simulink model "PID"  (R2024b)
settings: Solver=VariableStepAuto  StartTime=0.0  StopTime=t_sim  RelTol=1e-3
values from neighbouring files (symbols this model uses):
  Ax = [0 1; 0 0]    [Main_PID.m]
  Ay = [0 1; 0 0]    [Main_PID.m]
  b = 0.0245    [Main_PID.m]
  Bx = [0 Cx]'    [Main_PID.m]
  By = [0 Cy]'    [Main_PID.m]
  CCx = [1 0]    [Main_PID.m]
  CCy = [1 0]    [Main_PID.m]
  Cx = m*g*b/(m+J/r^2)/lx    (= 0.943269230769)    [Main_PID.m]
  Cy = m*g*b/(m+J/r^2)/ly    (= 1.1445)    [Main_PID.m]
  data_sys = [m r g J b lx ly]    [Main_PID.m]
  Dx = 0    [Main_PID.m]
  Dy = 0    [Main_PID.m]
  Kb_x = 0    [Main_PID.m]
  Kb_y = 0    [Main_PID.m]
  Kd_x = 3    [Main_PID.m]
  Kd_y = Kd_x/1.2    (= 2.5)    [Main_PID.m]
  Ki_x = 5    [Main_PID.m]
  Ki_y = Ki_x/1.2    (= 4.16666666667)    [Main_PID.m]
  Kp_x = 5    [Main_PID.m]
  Kp_y = Kp_x/1.2    (= 4.16666666667)    [Main_PID.m]
  lx = 0.182    [Main_PID.m]
  ly = 0.150    (= 0.15)    [Main_PID.m]
  N_x = 15    [Main_PID.m]
  N_y = 15    [Main_PID.m]
  ux_lim = 45    [Main_PID.m]
  uy_lim = 45    [Main_PID.m]
  x_ref = 0.05    [Main_PID.m]
  y_ref = 0.05    [Main_PID.m]
  zx0 = [x0 xp0]'    [Main_PID.m]
  zy0 = [y0 yp0]'    [Main_PID.m]
libraries: slpidlib x4
settings Model: Creator=nicvi  LastModifiedBy=nicvi

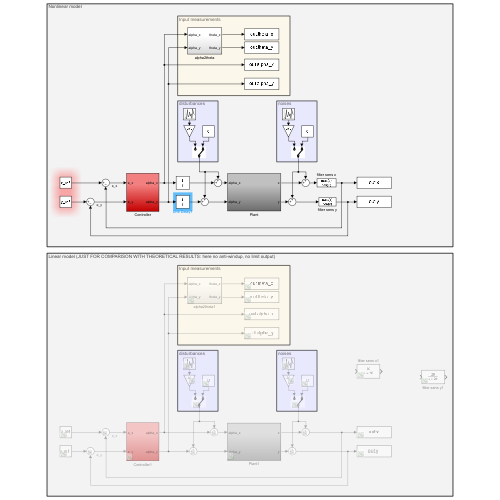
[thumbnail: Simulink's stored preview of the top-level diagram]
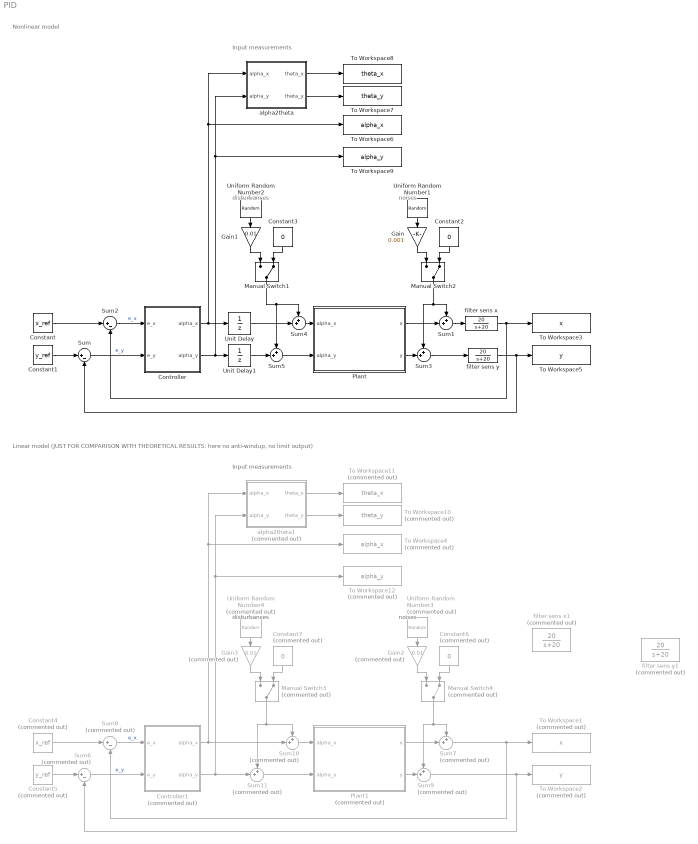
== system PID ==
  note: Nonlinear model
  note: noises
  note: Input measurements
  note: disturbances
  note: Linear model (JUST FOR COMPARISON WITH THEORETICAL RESULTS: here no anti-windup, no limit output)
  note: noises
  note: disturbances
  note: Input measurements
  Constant : Constant  Value=x_ref  SampleTime=-1
  Constant1 : Constant  Value=y_ref  SampleTime=-1
  Constant2 : Constant  Value=0
  Constant3 : Constant  Value=0
  Constant4 : Constant  Commented=on  Value=x_ref  SampleTime=-1
  Constant5 : Constant  Commented=on  Value=y_ref  SampleTime=-1
  Constant6 : Constant  Commented=on  Value=0
  Constant7 : Constant  Commented=on  Value=0
  Controller : Subsystem
  Controller1 : Subsystem  Commented=on
  Gain : Gain  Gain=0.001
  Gain1 : Gain  Gain=0.01
  Gain2 : Gain  Commented=on  Gain=0.01
  Gain3 : Gain  Commented=on  Gain=0.01
  Manual Switch1 : ManualSwitch  CurrentSetting=0
  Manual Switch2 : ManualSwitch  CurrentSetting=0
  Manual Switch3 : ManualSwitch  Commented=on  CurrentSetting=0
  Manual Switch4 : ManualSwitch  Commented=on  CurrentSetting=0
  Plant : Subsystem
  Plant1 : Subsystem  Commented=on
  Sum : Sum  Inputs=|+-
  Sum{1,3..5} (4 alike) : Sum  Inputs=++|
  Sum{7,9..11} (4 alike) : Sum  Commented=on  Inputs=++|
  Sum2 : Sum  Inputs=|+-
  Sum6 : Sum  Commented=on  Inputs=|+-
  Sum8 : Sum  Commented=on  Inputs=|+-
  To Workspace1 : ToWorkspace  Commented=on  VariableName=x  SampleTime=-1
      settings: Save2DSignal=2-D array (concatenate along first dimension)
  To Workspace10 : ToWorkspace  Commented=on  VariableName=theta_y  SampleTime=-1
      settings: Save2DSignal=2-D array (concatenate along first dimension)
  To Workspace11 : ToWorkspace  Commented=on  VariableName=theta_x  SampleTime=-1
      settings: Save2DSignal=2-D array (concatenate along first dimension)
  To Workspace12 : ToWorkspace  Commented=on  VariableName=alpha_y  SampleTime=-1
      settings: Save2DSignal=2-D array (concatenate along first dimension)
  To Workspace2 : ToWorkspace  Commented=on  VariableName=y  SampleTime=-1
      settings: Save2DSignal=2-D array (concatenate along first dimension)
  To Workspace3 : ToWorkspace  VariableName=x  SampleTime=-1
      settings: Save2DSignal=2-D array (concatenate along first dimension)
  To Workspace4 : ToWorkspace  Commented=on  VariableName=alpha_x  SampleTime=-1
      settings: Save2DSignal=2-D array (concatenate along first dimension)
  To Workspace5 : ToWorkspace  VariableName=y  SampleTime=-1
      settings: Save2DSignal=2-D array (concatenate along first dimension)
  To Workspace6 : ToWorkspace  VariableName=alpha_x  SampleTime=-1
      settings: Save2DSignal=2-D array (concatenate along first dimension)
  To Workspace7 : ToWorkspace  VariableName=theta_y  SampleTime=-1
      settings: Save2DSignal=2-D array (concatenate along first dimension)
  To Workspace8 : ToWorkspace  VariableName=theta_x  SampleTime=-1
      settings: Save2DSignal=2-D array (concatenate along first dimension)
  To Workspace9 : ToWorkspace  VariableName=alpha_y  SampleTime=-1
      settings: Save2DSignal=2-D array (concatenate along first dimension)
  Uniform Random Number1 : UniformRandomNumber  SampleTime=0.1
  Uniform Random Number2 : UniformRandomNumber  Minimum=5  Maximum=7  SampleTime=0.01
  Uniform Random Number3 : UniformRandomNumber  Commented=on  SampleTime=0.01
  Uniform Random Number4 : UniformRandomNumber  Commented=on  SampleTime=0.01
  Unit Delay : UnitDelay  SampleTime=0.08  HasFrameUpgradeWarning=on
  Unit Delay1 : UnitDelay  SampleTime=0.08  HasFrameUpgradeWarning=on
  alpha2theta : Subsystem
  alpha2theta1 : Subsystem  Commented=on
  filter sens x : TransferFcn  Numerator=[20]  Denominator=[1 20]
  filter sens x1 : TransferFcn  Commented=on  Numerator=[20]  Denominator=[1 20]
  filter sens y : TransferFcn  Numerator=[20]  Denominator=[1 20]
  filter sens y1 : TransferFcn  Commented=on  Numerator=[20]  Denominator=[1 20]
  wires:
  Constant/1 -> Sum2/1
  Constant1/1 -> Sum/1
  Sum2/1 -> Controller/1(e_x)  "e_x"
  Sum/1 -> Controller/2(e_y)  "e_y"
  Controller/1(alpha_x) -> Unit Delay/1, To Workspace6/1, alpha2theta/1(alpha_x)
  Controller/2(alpha_y) -> To Workspace9/1, alpha2theta/2(alpha_y), Unit Delay1/1
  alpha2theta/1(theta_x) -> To Workspace8/1
  alpha2theta/2(theta_y) -> To Workspace7/1
  Plant/2(y) -> Sum3/2
  Plant/1(x) -> Sum1/2
  Constant2/1 -> Manual Switch2/2
  Uniform Random Number1/1 -> Gain/1
  Gain/1 -> Manual Switch2/1
  Manual Switch2/1 -> Sum1/1, Sum3/1
  Manual Switch1/1 -> Sum5/1, Sum4/1
  Constant3/1 -> Manual Switch1/2
  Gain1/1 -> Manual Switch1/1
  Uniform Random Number2/1 -> Gain1/1
  Sum4/1 -> Plant/1(alpha_x)
  Sum5/1 -> Plant/2(alpha_y)
  Uniform Random Number3/1 -> Gain2/1
  Sum10/1 -> Plant1/1(alpha_x)
  Manual Switch3/1 -> Sum11/1, Sum10/1
  alpha2theta1/1(theta_x) -> To Workspace11/1
  Sum8/1 -> Controller1/1(e_x)  "e_x"
  Constant5/1 -> Sum6/1
  Controller1/2(alpha_y) -> Sum11/2, To Workspace12/1, alpha2theta1/2(alpha_y)
  Sum11/1 -> Plant1/2(alpha_y)
  Controller1/1(alpha_x) -> Sum10/2, To Workspace4/1, alpha2theta1/1(alpha_x)
  Constant4/1 -> Sum8/1
  Sum6/1 -> Controller1/2(e_y)  "e_y"
  Constant7/1 -> Manual Switch3/2
  Manual Switch4/1 -> Sum7/1, Sum9/1
  alpha2theta1/2(theta_y) -> To Workspace10/1
  Plant1/2(y) -> Sum9/2
  Sum9/1 -> To Workspace2/1, Sum6/2
  Gain2/1 -> Manual Switch4/1
  Gain3/1 -> Manual Switch3/1
  Uniform Random Number4/1 -> Gain3/1
  Constant6/1 -> Manual Switch4/2
  Sum7/1 -> To Workspace1/1, Sum8/2
  Plant1/1(x) -> Sum7/2
  Sum1/1 -> filter sens x/1
  Sum3/1 -> filter sens y/1
  filter sens x/1 -> To Workspace3/1, Sum2/2
  filter sens y/1 -> To Workspace5/1, Sum/2
  Unit Delay/1 -> Sum4/2
  Unit Delay1/1 -> Sum5/2

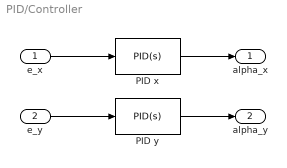
== system PID/Controller ==
  e_x : Inport
  e_y : Inport  Port=2
  PID x : slpidlib/PID Controller  Controller=PID  Form=Parallel  TimeDomain=Continuous-time  UseExternalTs=off  SampleTime=-1  IntegratorMethod=Forward Euler  FilterMethod=Forward Euler  ControllerParametersSource=internal  P=Kp_x  I=Ki_x  UseKiTs=off  D=Kd_x  UseExternalDerivativeSource=off  N=N_x  UseFilter=on  TunerSelectOption=Transfer Function Based (PID Tuner App)  InitialConditionSource=internal  InitialConditionForIntegrator=0  InitialConditionForFilter=0  DifferentiatorICPrevScaledInput=0  ExternalReset=none  TrackingMode=off  Kt=1  LimitOutput=on  SatLimitsSource=internal  UpperSaturationLimit=deg2rad(ux_lim)  LowerSaturationLimit=deg2rad(-ux_lim)  LinearizeAsGain=on  AntiWindupMode=back-calculation  Kb=Kb_x  LimitIntegrator=off  UpperIntegratorSaturationLimit=inf  LowerIntegratorSaturationLimit=-inf  POutMin=[]  POutMax=[]  IOutMin=[]  IOutMax=[]  DOutMin=[]  DOutMax=[]  NOutMin=[]  NOutMax=[]  SumOutMin=[]  SumOutMax=[]  SaturationOutMin=[]  SaturationOutMax=[]  PParamMin=[]  PParamMax=[]  IParamMin=[]  IParamMax=[]  DParamMin=[]  DParamMax=[]  NParamMin=[]  NParamMax=[]  KbParamMin=[]  KbParamMax=[]  KtParamMin=[]  KtParamMax=[]  KbOutMin=[]  KbOutMax=[]  KtOutMin=[]  KtOutMax=[]  IntegratorOutMin=[]  IntegratorOutMax=[]  FilterOutMin=[]  FilterOutMax=[]  SumI1OutMin=[]  SumI1OutMax=[]  SumI2OutMin=[]  SumI2OutMax=[]  SumI3OutMin=[]  SumI3OutMax=[]  SumI4OutMin=[]  SumI4OutMax=[]  SumDOutMin=[]  SumDOutMax=[]  DifferentiatorOutMin=[]  DifferentiatorOutMax=[]  FilterDiffOutCoefMin=[]  FilterDiffOutCoefMax=[]  ReciprocalOutMin=[]  ReciprocalOutMax=[]  SumDenOutMin=[]  SumDenOutMax=[]  SumNumOutMin=[]  SumNumOutMax=[]  DivideOutMin=[]  DivideOutMax=[]  UdiffTsProdOutMin=[]  UdiffTsProdOutMax=[]  NTsProdOutMin=[]  NTsProdOutMax=[]  UintegralTsProdOutMin=[]  UintegralTsProdOutMax=[]  UngainTsProdOutMin=[]  UngainTsProdOutMax=[]  ClampingZeroOutDataTypeStr=Inherit: Inherit via back propagation  ClampingZeroOutMin=[]  ClampingZeroOutMax=[]  FilterDenConstantOutDataTypeStr=Inherit: Inherit via back propagation  FilterDenConstantOutMin=[]  FilterDenConstantOutMax=[]  PCopyOutDataTypeStr=Inherit: Inherit via back propagation  PCopyOutMin=[]  PCopyOutMax=[]  NCopyOutDataTypeStr=Inherit: Inherit via back propagation  NCopyOutMin=[]  NCopyOutMax=[]  IntegratorContinuousStateAttributes=''  IntegratorStateMustResolveToSignalObject=off  IntegratorRTWStateStorageClass=Auto  FilterContinuousStateAttributes=''  FilterStateMustResolveToSignalObject=off  FilterRTWStateStorageClass=Auto  ParallelPVariant=InternalParameters  IdealPVariant=Disabled  IVariant=InternalParameters  DVariant=InternalParameters  IntegratorVariant=Continuous  SatVariant=Enabled  AWVariant=BackCalculation  PCopyVariant=Disabled  TRVariant=Disabled  FdbkBlocksVariant=Forward  IdealPFdbkVariant=Disabled  SatFdbkVariant=Disabled  DerivativeFilterVariant=ContFilter  NVariant=InternalParameters  NCopyVariant=Disabled  FilterICVariant=InternalICsFilter  IntegratorICVariant=InternalICs  ExternalResetVariant=Disabled  TRSumVariant=Passthrough  SumFdbkVariant=Disabled  SumVariant=Sum_PID  TsampFilterVariant=InternalTs  TsampNgainVariant=Passthrough  TsampIntegralVariant=Disabled_SignalSpec  ExternalSaturationOutDataTypeStr=Inherit: Same as second input  DerivativeSourceVariant=ErrorSignal  PreIntVariant=InternalPreInt
  PID y : slpidlib/PID Controller  Controller=PID  Form=Parallel  TimeDomain=Continuous-time  UseExternalTs=off  SampleTime=-1  IntegratorMethod=Forward Euler  FilterMethod=Forward Euler  ControllerParametersSource=internal  P=Kp_y  I=Ki_y  UseKiTs=off  D=Kd_y  UseExternalDerivativeSource=off  N=N_y  UseFilter=on  TunerSelectOption=Transfer Function Based (PID Tuner App)  InitialConditionSource=internal  InitialConditionForIntegrator=0  InitialConditionForFilter=0  DifferentiatorICPrevScaledInput=0  ExternalReset=none  TrackingMode=off  Kt=1  LimitOutput=on  SatLimitsSource=internal  UpperSaturationLimit=deg2rad(uy_lim)  LowerSaturationLimit=deg2rad(-uy_lim)  LinearizeAsGain=on  AntiWindupMode=back-calculation  Kb=Kb_y  LimitIntegrator=off  UpperIntegratorSaturationLimit=inf  LowerIntegratorSaturationLimit=-inf  POutMin=[]  POutMax=[]  IOutMin=[]  IOutMax=[]  DOutMin=[]  DOutMax=[]  NOutMin=[]  NOutMax=[]  SumOutMin=[]  SumOutMax=[]  SaturationOutMin=[]  SaturationOutMax=[]  PParamMin=[]  PParamMax=[]  IParamMin=[]  IParamMax=[]  DParamMin=[]  DParamMax=[]  NParamMin=[]  NParamMax=[]  KbParamMin=[]  KbParamMax=[]  KtParamMin=[]  KtParamMax=[]  KbOutMin=[]  KbOutMax=[]  KtOutMin=[]  KtOutMax=[]  IntegratorOutMin=[]  IntegratorOutMax=[]  FilterOutMin=[]  FilterOutMax=[]  SumI1OutMin=[]  SumI1OutMax=[]  SumI2OutMin=[]  SumI2OutMax=[]  SumI3OutMin=[]  SumI3OutMax=[]  SumI4OutMin=[]  SumI4OutMax=[]  SumDOutMin=[]  SumDOutMax=[]  DifferentiatorOutMin=[]  DifferentiatorOutMax=[]  FilterDiffOutCoefMin=[]  FilterDiffOutCoefMax=[]  ReciprocalOutMin=[]  ReciprocalOutMax=[]  SumDenOutMin=[]  SumDenOutMax=[]  SumNumOutMin=[]  SumNumOutMax=[]  DivideOutMin=[]  DivideOutMax=[]  UdiffTsProdOutMin=[]  UdiffTsProdOutMax=[]  NTsProdOutMin=[]  NTsProdOutMax=[]  UintegralTsProdOutMin=[]  UintegralTsProdOutMax=[]  UngainTsProdOutMin=[]  UngainTsProdOutMax=[]  ClampingZeroOutDataTypeStr=Inherit: Inherit via back propagation  ClampingZeroOutMin=[]  ClampingZeroOutMax=[]  FilterDenConstantOutDataTypeStr=Inherit: Inherit via back propagation  FilterDenConstantOutMin=[]  FilterDenConstantOutMax=[]  PCopyOutDataTypeStr=Inherit: Inherit via back propagation  PCopyOutMin=[]  PCopyOutMax=[]  NCopyOutDataTypeStr=Inherit: Inherit via back propagation  NCopyOutMin=[]  NCopyOutMax=[]  IntegratorContinuousStateAttributes=''  IntegratorStateMustResolveToSignalObject=off  IntegratorRTWStateStorageClass=Auto  FilterContinuousStateAttributes=''  FilterStateMustResolveToSignalObject=off  FilterRTWStateStorageClass=Auto  ParallelPVariant=InternalParameters  IdealPVariant=Disabled  IVariant=InternalParameters  DVariant=InternalParameters  IntegratorVariant=Continuous  SatVariant=Enabled  AWVariant=BackCalculation  PCopyVariant=Disabled  TRVariant=Disabled  FdbkBlocksVariant=Forward  IdealPFdbkVariant=Disabled  SatFdbkVariant=Disabled  DerivativeFilterVariant=ContFilter  NVariant=InternalParameters  NCopyVariant=Disabled  FilterICVariant=InternalICsFilter  IntegratorICVariant=InternalICs  ExternalResetVariant=Disabled  TRSumVariant=Passthrough  SumFdbkVariant=Disabled  SumVariant=Sum_PID  TsampFilterVariant=InternalTs  TsampNgainVariant=Passthrough  TsampIntegralVariant=Disabled_SignalSpec  ExternalSaturationOutDataTypeStr=Inherit: Same as second input  DerivativeSourceVariant=ErrorSignal  PreIntVariant=InternalPreInt
  alpha_x : Outport
  alpha_y : Outport  Port=2
  wires:
  PID y/1 -> alpha_y/1
  e_y/1 -> PID y/1
  e_x/1 -> PID x/1
  PID x/1 -> alpha_x/1

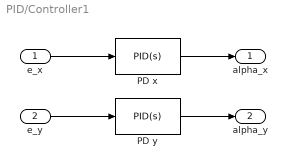
== system PID/Controller1 ==
  e_x : Inport
  e_y : Inport  Port=2
  PD x : slpidlib/PID Controller  Controller=PID  Form=Parallel  TimeDomain=Continuous-time  UseExternalTs=off  SampleTime=-1  IntegratorMethod=Forward Euler  FilterMethod=Forward Euler  ControllerParametersSource=internal  P=Kp_x  I=Ki_x  UseKiTs=off  D=Kd_x  UseExternalDerivativeSource=off  N=N_x  UseFilter=on  TunerSelectOption=Transfer Function Based (PID Tuner App)  InitialConditionSource=internal  InitialConditionForIntegrator=0  InitialConditionForFilter=0  DifferentiatorICPrevScaledInput=0  ExternalReset=none  TrackingMode=off  Kt=1  LimitOutput=on  SatLimitsSource=internal  UpperSaturationLimit=deg2rad(ux_lim)  LowerSaturationLimit=deg2rad(-ux_lim)  LinearizeAsGain=on  AntiWindupMode=back-calculation  Kb=Kb_x  LimitIntegrator=off  UpperIntegratorSaturationLimit=inf  LowerIntegratorSaturationLimit=-inf  POutMin=[]  POutMax=[]  IOutMin=[]  IOutMax=[]  DOutMin=[]  DOutMax=[]  NOutMin=[]  NOutMax=[]  SumOutMin=[]  SumOutMax=[]  SaturationOutMin=[]  SaturationOutMax=[]  PParamMin=[]  PParamMax=[]  IParamMin=[]  IParamMax=[]  DParamMin=[]  DParamMax=[]  NParamMin=[]  NParamMax=[]  KbParamMin=[]  KbParamMax=[]  KtParamMin=[]  KtParamMax=[]  KbOutMin=[]  KbOutMax=[]  KtOutMin=[]  KtOutMax=[]  IntegratorOutMin=[]  IntegratorOutMax=[]  FilterOutMin=[]  FilterOutMax=[]  SumI1OutMin=[]  SumI1OutMax=[]  SumI2OutMin=[]  SumI2OutMax=[]  SumI3OutMin=[]  SumI3OutMax=[]  SumI4OutMin=[]  SumI4OutMax=[]  SumDOutMin=[]  SumDOutMax=[]  DifferentiatorOutMin=[]  DifferentiatorOutMax=[]  FilterDiffOutCoefMin=[]  FilterDiffOutCoefMax=[]  ReciprocalOutMin=[]  ReciprocalOutMax=[]  SumDenOutMin=[]  SumDenOutMax=[]  SumNumOutMin=[]  SumNumOutMax=[]  DivideOutMin=[]  DivideOutMax=[]  UdiffTsProdOutMin=[]  UdiffTsProdOutMax=[]  NTsProdOutMin=[]  NTsProdOutMax=[]  UintegralTsProdOutMin=[]  UintegralTsProdOutMax=[]  UngainTsProdOutMin=[]  UngainTsProdOutMax=[]  ClampingZeroOutDataTypeStr=Inherit: Inherit via back propagation  ClampingZeroOutMin=[]  ClampingZeroOutMax=[]  FilterDenConstantOutDataTypeStr=Inherit: Inherit via back propagation  FilterDenConstantOutMin=[]  FilterDenConstantOutMax=[]  PCopyOutDataTypeStr=Inherit: Inherit via back propagation  PCopyOutMin=[]  PCopyOutMax=[]  NCopyOutDataTypeStr=Inherit: Inherit via back propagation  NCopyOutMin=[]  NCopyOutMax=[]  IntegratorContinuousStateAttributes=''  IntegratorStateMustResolveToSignalObject=off  IntegratorRTWStateStorageClass=Auto  FilterContinuousStateAttributes=''  FilterStateMustResolveToSignalObject=off  FilterRTWStateStorageClass=Auto  ParallelPVariant=InternalParameters  IdealPVariant=Disabled  IVariant=InternalParameters  DVariant=InternalParameters  IntegratorVariant=Continuous  SatVariant=Enabled  AWVariant=BackCalculation  PCopyVariant=Disabled  TRVariant=Disabled  FdbkBlocksVariant=Forward  IdealPFdbkVariant=Disabled  SatFdbkVariant=Disabled  DerivativeFilterVariant=ContFilter  NVariant=InternalParameters  NCopyVariant=Disabled  FilterICVariant=InternalICsFilter  IntegratorICVariant=InternalICs  ExternalResetVariant=Disabled  TRSumVariant=Passthrough  SumFdbkVariant=Disabled  SumVariant=Sum_PID  TsampFilterVariant=InternalTs  TsampNgainVariant=Passthrough  TsampIntegralVariant=Disabled_SignalSpec  ExternalSaturationOutDataTypeStr=Inherit: Same as second input  DerivativeSourceVariant=ErrorSignal  PreIntVariant=InternalPreInt
  PD y : slpidlib/PID Controller  Controller=PID  Form=Parallel  TimeDomain=Continuous-time  UseExternalTs=off  SampleTime=-1  IntegratorMethod=Forward Euler  FilterMethod=Forward Euler  ControllerParametersSource=internal  P=Kp_y  I=Ki_y  UseKiTs=off  D=Kd_y  UseExternalDerivativeSource=off  N=N_y  UseFilter=on  TunerSelectOption=Transfer Function Based (PID Tuner App)  InitialConditionSource=internal  InitialConditionForIntegrator=0  InitialConditionForFilter=0  DifferentiatorICPrevScaledInput=0  ExternalReset=none  TrackingMode=off  Kt=1  LimitOutput=on  SatLimitsSource=internal  UpperSaturationLimit=deg2rad(uy_lim)  LowerSaturationLimit=deg2rad(-uy_lim)  LinearizeAsGain=on  AntiWindupMode=back-calculation  Kb=Kb_y  LimitIntegrator=off  UpperIntegratorSaturationLimit=inf  LowerIntegratorSaturationLimit=-inf  POutMin=[]  POutMax=[]  IOutMin=[]  IOutMax=[]  DOutMin=[]  DOutMax=[]  NOutMin=[]  NOutMax=[]  SumOutMin=[]  SumOutMax=[]  SaturationOutMin=[]  SaturationOutMax=[]  PParamMin=[]  PParamMax=[]  IParamMin=[]  IParamMax=[]  DParamMin=[]  DParamMax=[]  NParamMin=[]  NParamMax=[]  KbParamMin=[]  KbParamMax=[]  KtParamMin=[]  KtParamMax=[]  KbOutMin=[]  KbOutMax=[]  KtOutMin=[]  KtOutMax=[]  IntegratorOutMin=[]  IntegratorOutMax=[]  FilterOutMin=[]  FilterOutMax=[]  SumI1OutMin=[]  SumI1OutMax=[]  SumI2OutMin=[]  SumI2OutMax=[]  SumI3OutMin=[]  SumI3OutMax=[]  SumI4OutMin=[]  SumI4OutMax=[]  SumDOutMin=[]  SumDOutMax=[]  DifferentiatorOutMin=[]  DifferentiatorOutMax=[]  FilterDiffOutCoefMin=[]  FilterDiffOutCoefMax=[]  ReciprocalOutMin=[]  ReciprocalOutMax=[]  SumDenOutMin=[]  SumDenOutMax=[]  SumNumOutMin=[]  SumNumOutMax=[]  DivideOutMin=[]  DivideOutMax=[]  UdiffTsProdOutMin=[]  UdiffTsProdOutMax=[]  NTsProdOutMin=[]  NTsProdOutMax=[]  UintegralTsProdOutMin=[]  UintegralTsProdOutMax=[]  UngainTsProdOutMin=[]  UngainTsProdOutMax=[]  ClampingZeroOutDataTypeStr=Inherit: Inherit via back propagation  ClampingZeroOutMin=[]  ClampingZeroOutMax=[]  FilterDenConstantOutDataTypeStr=Inherit: Inherit via back propagation  FilterDenConstantOutMin=[]  FilterDenConstantOutMax=[]  PCopyOutDataTypeStr=Inherit: Inherit via back propagation  PCopyOutMin=[]  PCopyOutMax=[]  NCopyOutDataTypeStr=Inherit: Inherit via back propagation  NCopyOutMin=[]  NCopyOutMax=[]  IntegratorContinuousStateAttributes=''  IntegratorStateMustResolveToSignalObject=off  IntegratorRTWStateStorageClass=Auto  FilterContinuousStateAttributes=''  FilterStateMustResolveToSignalObject=off  FilterRTWStateStorageClass=Auto  ParallelPVariant=InternalParameters  IdealPVariant=Disabled  IVariant=InternalParameters  DVariant=InternalParameters  IntegratorVariant=Continuous  SatVariant=Enabled  AWVariant=BackCalculation  PCopyVariant=Disabled  TRVariant=Disabled  FdbkBlocksVariant=Forward  IdealPFdbkVariant=Disabled  SatFdbkVariant=Disabled  DerivativeFilterVariant=ContFilter  NVariant=InternalParameters  NCopyVariant=Disabled  FilterICVariant=InternalICsFilter  IntegratorICVariant=InternalICs  ExternalResetVariant=Disabled  TRSumVariant=Passthrough  SumFdbkVariant=Disabled  SumVariant=Sum_PID  TsampFilterVariant=InternalTs  TsampNgainVariant=Passthrough  TsampIntegralVariant=Disabled_SignalSpec  ExternalSaturationOutDataTypeStr=Inherit: Same as second input  DerivativeSourceVariant=ErrorSignal  PreIntVariant=InternalPreInt
  alpha_x : Outport
  alpha_y : Outport  Port=2
  wires:
  PD y/1 -> alpha_y/1
  e_y/1 -> PD y/1
  e_x/1 -> PD x/1
  PD x/1 -> alpha_x/1

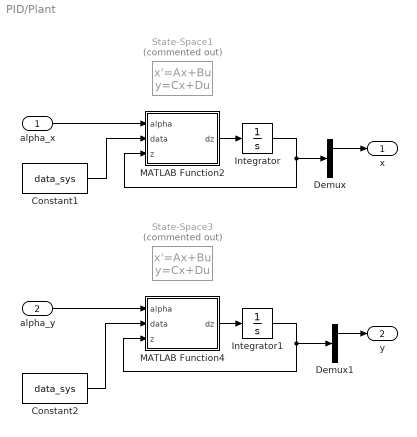
== system PID/Plant ==
  alpha_x : Inport
  alpha_y : Inport  Port=2
  Constant1 : Constant  Value=data_sys
  Constant2 : Constant  Value=data_sys
  Demux : Demux  Outputs=2
  Demux1 : Demux  Outputs=2
  Integrator : Integrator  InitialCondition=zx0
  Integrator1 : Integrator  InitialCondition=zy0
  MATLAB Function2 : MATLAB Function  TreatAsAtomicUnit=on
  MATLAB Function4 : MATLAB Function  TreatAsAtomicUnit=on
  State-Space1 : StateSpace  Commented=on  A=Ax  B=Bx  C=Cx  D=Dx  InitialCondition=zx0
  State-Space3 : StateSpace  Commented=on  A=Ay  B=By  C=Cy  D=Dy  InitialCondition=zy0
  x : Outport
  y : Outport  Port=2
  wires:
  alpha_y/1 -> MATLAB Function4/1(alpha)
  alpha_x/1 -> MATLAB Function2/1(alpha)
  Constant1/1 -> MATLAB Function2/2(data)
  MATLAB Function2/1(dz) -> Integrator/1
  Integrator/1 -> MATLAB Function2/3(z), Demux/1
  MATLAB Function4/1(dz) -> Integrator1/1
  Constant2/1 -> MATLAB Function4/2(data)
  Demux/1 -> x/1
  Demux1/1 -> y/1
  Integrator1/1 -> MATLAB Function4/3(z), Demux1/1

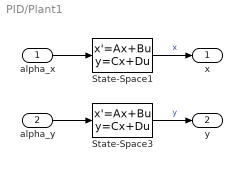
== system PID/Plant1 ==
  alpha_x : Inport
  alpha_y : Inport  Port=2
  State-Space1 : StateSpace  A=Ax  B=Bx  C=CCx  D=Dx  InitialCondition=zx0
  State-Space3 : StateSpace  A=Ay  B=By  C=CCy  D=Dy  InitialCondition=zy0
  x : Outport
  y : Outport  Port=2
  wires:
  alpha_y/1 -> State-Space3/1
  alpha_x/1 -> State-Space1/1
  State-Space1/1 -> x/1  "x"
  State-Space3/1 -> y/1  "y"

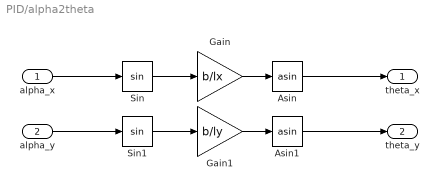
== system PID/alpha2theta ==
  alpha_x : Inport
  alpha_y : Inport  Port=2
  Asin : Trigonometry  Operator=asin
  Asin1 : Trigonometry  Operator=asin
  Gain : Gain  Gain=b/lx
  Gain1 : Gain  Gain=b/ly
  Sin : Trigonometry
  Sin1 : Trigonometry
  theta_x : Outport
  theta_y : Outport  Port=2
  wires:
  Gain/1 -> Asin/1
  Sin1/1 -> Gain1/1
  alpha_y/1 -> Sin1/1
  Sin/1 -> Gain/1
  Asin1/1 -> theta_y/1
  Gain1/1 -> Asin1/1
  Asin/1 -> theta_x/1
  alpha_x/1 -> Sin/1

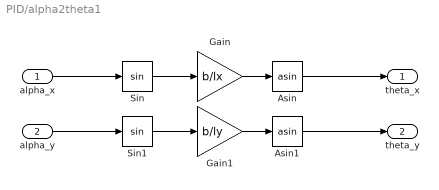
== system PID/alpha2theta1 ==
  alpha_x : Inport
  alpha_y : Inport  Port=2
  Asin : Trigonometry  Operator=asin
  Asin1 : Trigonometry  Operator=asin
  Gain : Gain  Gain=b/lx
  Gain1 : Gain  Gain=b/ly
  Sin : Trigonometry
  Sin1 : Trigonometry
  theta_x : Outport
  theta_y : Outport  Port=2
  wires:
  Gain/1 -> Asin/1
  Sin1/1 -> Gain1/1
  alpha_y/1 -> Sin1/1
  Sin/1 -> Gain/1
  Asin1/1 -> theta_y/1
  Gain1/1 -> Asin1/1
  Asin/1 -> theta_x/1
  alpha_x/1 -> Sin/1

== matlab function PID/Plant/MATLAB Function4 ==
  data: alpha input; dz output; data input; z input
function dz  = fcn(alpha,data,z)

m=data(1);
r=data(2);
g=data(3);
J=data(4);
b=data(5);
ly=data(7);

Cy=m*g*b/(m+J/r^2)/ly;

dz=zeros(2,1);
dz(1)=z(2);
dz(2)=Cy*sin(alpha);

end

== matlab function PID/Plant/MATLAB Function2 ==
  data: alpha input; dz output; data input; z input
function dz  = fcn(alpha,data,z)

m=data(1);
r=data(2);
g=data(3);
J=data(4);
b=data(5);
lx=data(6);

Cx=m*g*b/(m+J/r^2)/lx;

dz=zeros(2,1);
dz(1)=z(2);
dz(2)=Cx*sin(alpha);

end
